simulink model "lr41_21"  (R2022b)
settings: Solver=VariableStepAuto  StartTime=0.0  StopTime=200  MaxStep=0.01  MinStep=0.0001  RelTol=1e-3
InitFcn:
  | k0=6;
  | a0=-3;
  | a1=-4;
  | b0=2;
  | km0=12;
  | km1=36;
  | kg0=0.09; kg1=0.6;
  | A = [5 -4; 9 -1];
  | b = [0;6];
  | C = [1 0];
  | 
  | A0g = [0 1; -kg0 -kg1];
  | b0g=[0;1];
  | 
  | N = [0 0; 1 0];
  | Ad = [0 1; -256 -32];
  | H = [1 0];
  | M = lyap(A, -Ad, -b*H);
  | K=H*inv(M);
  | Am=A-b*K;
settings Model: Creator=thege  LastModifiedBy=Dimuss
settings DebuggingCC: UnconnectedInputMsg=warning  UnconnectedOutputMsg=warning  UnconnectedLineMsg=warning
settings ModelReferenceCC: EnableRefExpFcnMdlSchedulingChecks=on
settings RTWCC: DLArmComputeVersion=19.05

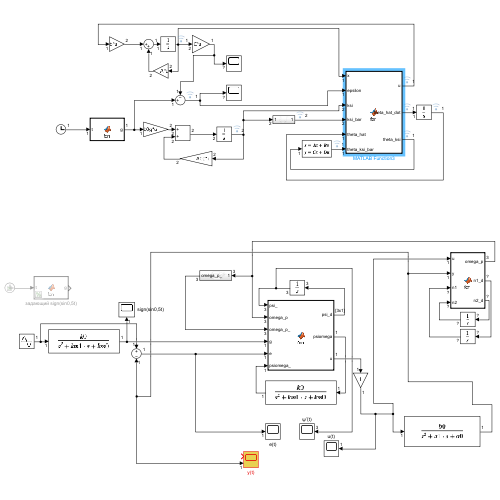
[thumbnail: Simulink's stored preview of the top-level diagram]
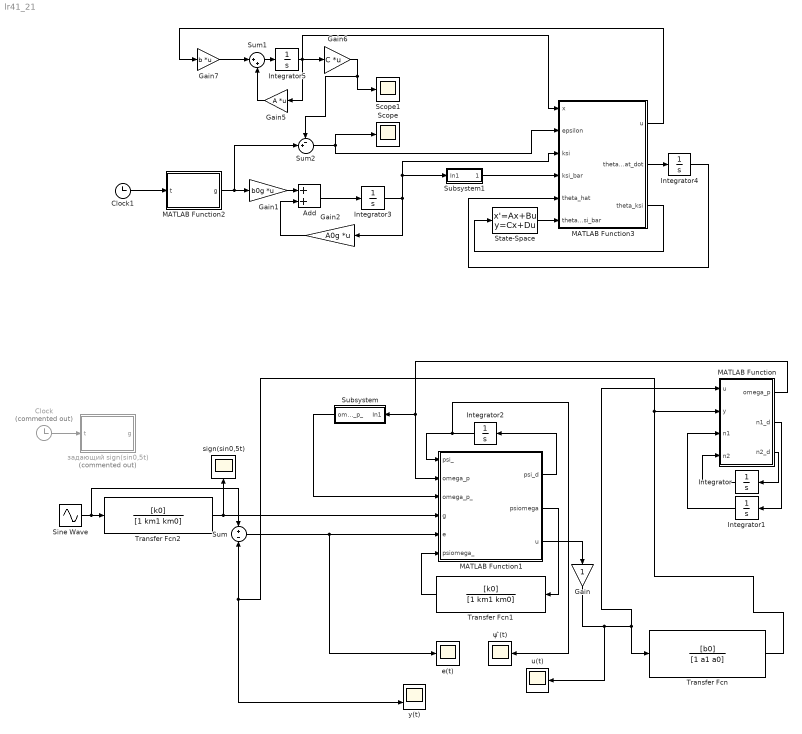
== system lr41_21 ==
  Add : Sum
  Clock : Clock  Commented=on
  Clock1 : Clock
  Gain : Gain
  Gain1 : Gain  Gain=b0g  Multiplication=Matrix(K*u)
  Gain2 : Gain  Gain=A0g  Multiplication=Matrix(K*u)
  Gain5 : Gain  Gain=A  Multiplication=Matrix(K*u)
  Gain6 : Gain  Gain=C  Multiplication=Matrix(K*u)
  Gain7 : Gain  Gain=b  Multiplication=Matrix(K*u)
  Integrator{,1,3..5} (5 alike) : Integrator
  Integrator2 : Integrator  InitialCondition=[0 0 0]'
  MATLAB Function : MATLAB Function  TreatAsAtomicUnit=on
  MATLAB Function1 : MATLAB Function  TreatAsAtomicUnit=on
  MATLAB Function2 : MATLAB Function  TreatAsAtomicUnit=on
  MATLAB Function3 : MATLAB Function  TreatAsAtomicUnit=on
  Scope : Scope
  Scope1 : Scope
  Sine Wave : Sin  SampleTime=0
  State-Space : StateSpace  A=Am  B=b  C=C  D=0  InitialCondition=0
  Subsystem : Subsystem
  Subsystem1 : Subsystem
  Sum : Sum  Inputs=+-
  Sum1 : Sum  Inputs=|++
  Sum2 : Sum  Inputs=-+|
  Transfer Fcn : TransferFcn  Numerator=[b0]  Denominator=[1 a1 a0]
  Transfer Fcn1 : TransferFcn  Numerator=[k0]  Denominator=[1 km1 km0]
  Transfer Fcn2 : TransferFcn  Numerator=[k0]  Denominator=[1 km1 km0]
  e(t) : Scope
  sign(sin0,5t) : Scope
  u(t) : Scope
  y(t) : Scope  NumInputPorts=2
  ψ ̂(t) : Scope
  задающий sign(sin0,5t) : MATLAB Function  Commented=on  TreatAsAtomicUnit=on
  wires:
  Clock/1 -> задающий sign(sin0,5t)/1(t)
  Transfer Fcn/1 -> Sum/2, y(t)/2, MATLAB Function/2(y)
  Sum/1 -> e(t)/1, MATLAB Function1/5(e)
  MATLAB Function/3(n2_d) -> Integrator/1
  Integrator/1 -> MATLAB Function/4(n2)
  MATLAB Function/2(n1_d) -> Integrator1/1
  Integrator1/1 -> MATLAB Function/3(n1)
  MATLAB Function1/2(psiomega) -> Transfer Fcn1/1
  Transfer Fcn1/1 -> MATLAB Function1/6(psiomega_)
  Gain/1 -> u(t)/1, Transfer Fcn/1, MATLAB Function/1(u)
  MATLAB Function1/3(u) -> Gain/1
  MATLAB Function1/1(psi_d) -> Integrator2/1
  Integrator2/1 -> MATLAB Function1/1(psi_), ψ ̂(t)/1
  MATLAB Function/1(omega_p) -> MATLAB Function1/2(omega_p), Subsystem/1(In1)
  Subsystem/1(omega_p_) -> MATLAB Function1/3(omega_p_)
  Sine Wave/1 -> Sum/1, Transfer Fcn2/1
  Transfer Fcn2/1 -> sign(sin0,5t)/1, MATLAB Function1/4(g)
  Gain6/1 -> Sum2/1, Scope1/1
  Integrator5/1 -> Gain5/1, MATLAB Function3/1(x), Gain6/1
  Gain5/1 -> Sum1/2
  Gain7/1 -> Sum1/1
  MATLAB Function3/1(u) -> Gain7/1
  Integrator4/1 -> MATLAB Function3/5(theta_hat)
  State-Space/1 -> MATLAB Function3/6(theta_ksi_bar)
  Sum1/1 -> Integrator5/1
  MATLAB Function2/1(g) -> Sum2/2, Gain1/1
  Gain1/1 -> Add/1
  Gain2/1 -> Add/2
  Add/1 -> Integrator3/1
  MATLAB Function3/3(theta_ksi) -> State-Space/1
  Clock1/1 -> MATLAB Function2/1(t)
  MATLAB Function3/2(theta_hat_dot) -> Integrator4/1
  Integrator3/1 -> MATLAB Function3/3(ksi), Subsystem1/1(In1), Gain2/1
  Subsystem1/1(Out1) -> MATLAB Function3/4(ksi_bar)
  Sum2/1 -> MATLAB Function3/2(epsilon), Scope/1

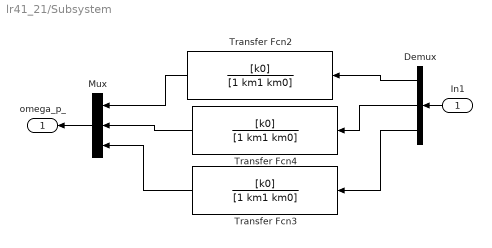
== system lr41_21/Subsystem ==
  In1 : Inport
  Demux : Demux  Outputs=3
  Mux : Mux  Inputs=3
  Transfer Fcn2 : TransferFcn  Numerator=[k0]  Denominator=[1 km1 km0]
  Transfer Fcn3 : TransferFcn  Numerator=[k0]  Denominator=[1 km1 km0]
  Transfer Fcn4 : TransferFcn  Numerator=[k0]  Denominator=[1 km1 km0]
  omega_p_ : Outport
  wires:
  Demux/2 -> Transfer Fcn4/1
  Demux/1 -> Transfer Fcn2/1
  Transfer Fcn4/1 -> Mux/2
  Demux/3 -> Transfer Fcn3/1
  Transfer Fcn2/1 -> Mux/1
  Mux/1 -> omega_p_/1
  In1/1 -> Demux/1
  Transfer Fcn3/1 -> Mux/3

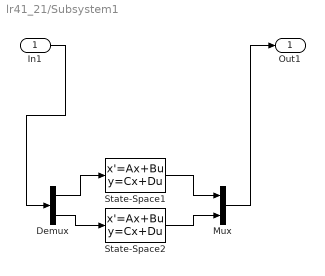
== system lr41_21/Subsystem1 ==
  In1 : Inport
  Demux : Demux  Outputs=2
  Mux : Mux  Inputs=2
  State-Space1 : StateSpace  A=Am  B=b  C=C  D=0  InitialCondition=0
  State-Space2 : StateSpace  A=Am  B=b  C=C  D=0  InitialCondition=0
  Out1 : Outport
  wires:
  Mux/1 -> Out1/1
  State-Space1/1 -> Mux/1
  Demux/1 -> State-Space1/1
  Demux/2 -> State-Space2/1
  In1/1 -> Demux/1
  State-Space2/1 -> Mux/2

== matlab function lr41_21/MATLAB Function1 ==
  data: psi_ input; psi_d output; psiomega output; omega_p input; omega_p_ input; g input; e input; psiomega_ input; u output; b0 parameter; k0 parameter
function [psi_d,psiomega,u]=fcn(psi_,omega_p,omega_p_,g,e,psiomega_, b0, k0)
psiomega=psi_'*omega_p;
e_=e-psi_'*omega_p_+psiomega_;
g1=0.1;
psi_d=g1*omega_p_*e_/(1+omega_p_'*omega_p_);
u=(psi_'*omega_p+k0*g)/b0;

== matlab function lr41_21/MATLAB Function ==
  data: u input; omega_p output; y input; n1 input; n2 input; n1_d output; n2_d output; k0 parameter
function [omega_p,n1_d,n2_d]=fcn(u,y,n1,n2, k0)
n1_d=-k0*n1+u;
n2_d=-k0*n2+y;
omega=[n1',n2',y]';
omega_p=-omega;

== matlab function lr41_21/задающий sign(sin0,5t) ==
  data: t input; g output
function g = fcn(t)
%g=2*sign(cos (t));
g = sign(sin(0.5*t));

== matlab function lr41_21/MATLAB Function2 ==
  data: t input; g output
function g = fcn(t)

g = 3*cos(4*t);

== matlab function lr41_21/MATLAB Function3 ==
  data: x input; epsilon input; ksi input; ksi_bar input; u output; theta_hat input; theta_hat_dot output; theta_ksi output; theta_ksi_bar input; K parameter
function [u, theta_hat_dot, theta_ksi] = fcn(x, epsilon, ksi, ksi_bar, theta_hat, theta_ksi_bar, K)

gamma=10;
theta_ksi=theta_hat'*ksi;
epsilon_hat=epsilon-theta_hat'*ksi_bar+theta_ksi_bar;
theta_hat_dot=gamma*ksi_bar*epsilon_hat;
u=-K*x+theta_hat'*ksi;
